simulink model "antifurto"  (Simulink 10.0)
settings: Solver=ode4  StartTime=0.0  StopTime=0  FixedStep=1e-4  RelTol=1e-5  EnableMultiTasking=on
settings Model: Creator=prof. G. Celentano  LastModifiedBy=giuseppericcio  ExtModeTrigMode=oneshot  ExtModeArmWhenConnect=off
settings DataIOCC: SignalLoggingSaveFormat=ModelDataLogs  SignalLoggingName=sigsOut
settings OptimizationCC: BooleanDataType=off  ExpressionDepthLimit=2147483647  InitFltsAndDblsToZero=on
settings DebuggingCC: SaveWithParameterizedLinksMsg=none  SignalResolutionControl=TryResolveAllWithWarning  MultiTaskDSMMsg=warning  MultiTaskCondExecSysMsg=none  FcnCallInpInsideContextMsg=warning  StateNameClashWarn=warning
settings HardwareCC: TargetUnknown=on
settings GRTTargetCC: TargetFcnLib=ansi_tfl_tmw.mat

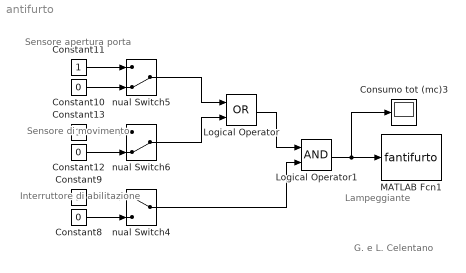
== system antifurto ==
  note: Interruttore di abilitazione
  note: Sensore apertura porta
  note: Sensore di movimento
  note: Lampeggiante
  note: G. e L. Celentano
  Constant10 : Constant  Value=0
  Constant11 : Constant
  Constant12 : Constant  Value=0
  Constant13 : Constant
  Constant8 : Constant  Value=0
  Constant9 : Constant
  Consumo tot (mc)3 : Display
  Logical Operator : Logic  Operator=OR
  Logical Operator1 : Logic
  MATLAB Fcn1 : MATLABFcn  MATLABFcn=fantifurto  OutputDimensions=0
  nual Switch4 : ManualSwitch
  nual Switch5 : ManualSwitch  CurrentSetting=0
  nual Switch6 : ManualSwitch  CurrentSetting=0
  wires:
  Logical Operator/1 -> Logical Operator1/1
  Constant13/1 -> nual Switch6/1
  Constant12/1 -> nual Switch6/2
  Constant9/1 -> nual Switch4/1
  Constant8/1 -> nual Switch4/2
  Constant11/1 -> nual Switch5/1
  Constant10/1 -> nual Switch5/2
  nual Switch6/1 -> Logical Operator/2
  nual Switch5/1 -> Logical Operator/1
  nual Switch4/1 -> Logical Operator1/2
  Logical Operator1/1 -> MATLAB Fcn1/1, Consumo tot (mc)3/1
